simulink model "untitled"  (R2020a)
settings: Solver=VariableStepAuto  StartTime=0.0  StopTime=100  RelTol=1e-3
settings Model: Creator=nartc  LastModifiedBy=nartc

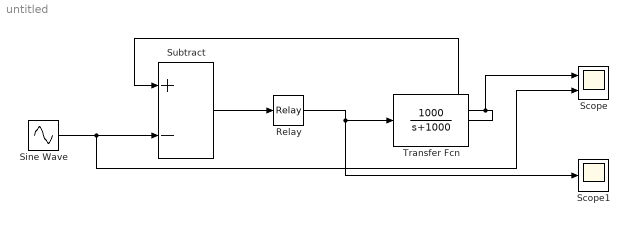
== system untitled ==
  Relay : Relay  OnSwitchValue=1  OffSwitchValue=-1  OnOutputValue=-12  OffOutputValue=12
  Scope : Scope  NumInputPorts=2
  Scope1 : Scope
  Sine Wave : Sin  Amplitude=10  Frequency=2*pi*[.01]  SampleTime=0
  Subtract : Sum  Inputs=+-
  Transfer Fcn : TransferFcn  Numerator=[1000]  Denominator=[1 1000]
  wires:
  Subtract/1 -> Relay/1
  Relay/1 -> Scope1/1, Transfer Fcn/1
  Sine Wave/1 -> Scope/2, Subtract/2
  Transfer Fcn/1 -> Subtract/1, Scope/1
